simulink model "DOF4_model"  (R2022b)
settings: Solver=VariableStepAuto  StartTime=0.0  StopTime=10.0  RelTol=1e-3
values from neighbouring files (symbols this model uses):
  cdamper = 1500    [Quarter_car_model_parameters.m]
  F0 = 3924    [Quarter_car_model_parameters.m]
  g = 9.81    [Longitudinal_braking_parameters.m]    (also in Longitudinal_driving_parameters.m; Quarter_car_model_parameters.m)
  kspring = 35500    [Quarter_car_model_parameters.m]
  ktyre = 300000    [Quarter_car_model_parameters.m]
  ms = 400    [Quarter_car_model_parameters.m]
  mus = 30    [Quarter_car_model_parameters.m]
  z0tyre = (ms+mus) * g/ktyre    (= 0.014061)    [Quarter_car_model_parameters.m]
settings Model: Creator=webstert  LastModifiedBy=webstert

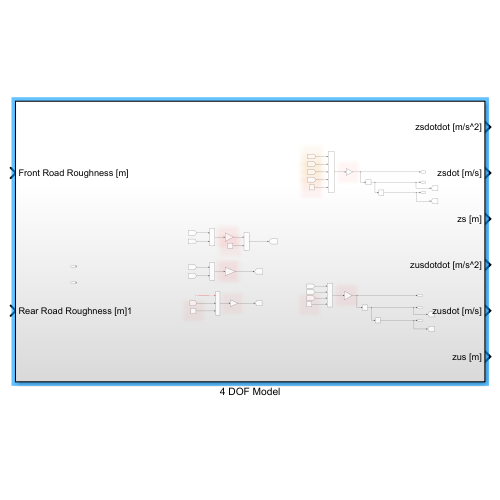
[thumbnail: Simulink's stored preview of the top-level diagram]
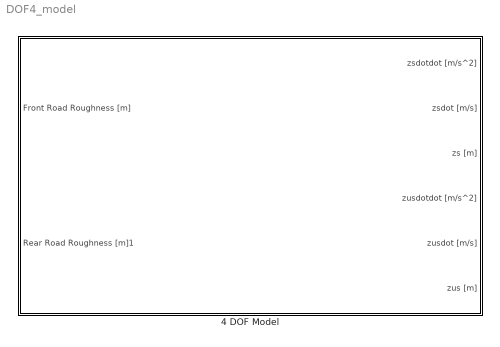
== system DOF4_model ==
  4 DOF Model : Subsystem

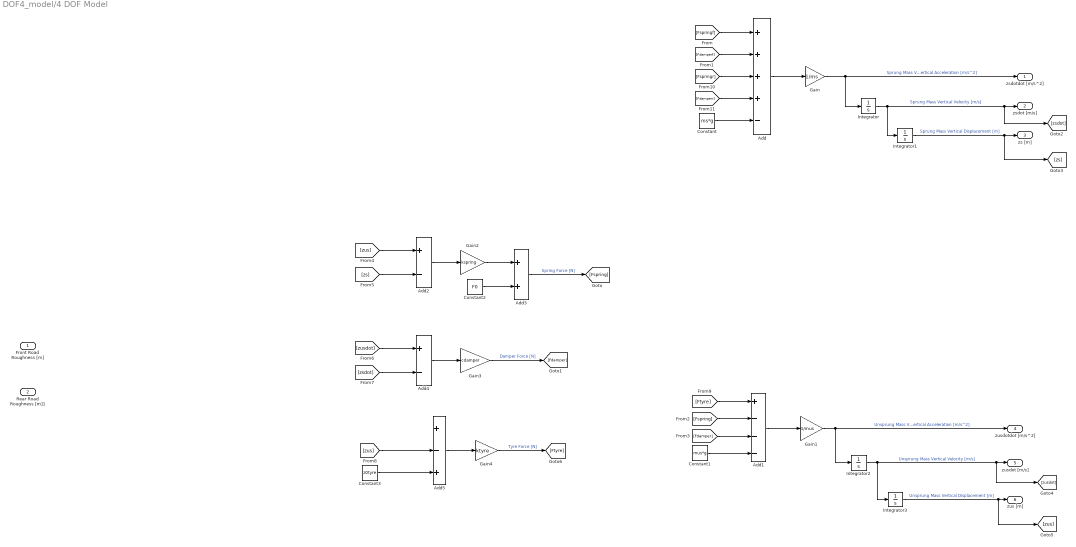
== system DOF4_model/4 DOF Model ==
  Front Road Roughness [m] : Inport
  Rear Road Roughness [m]1 : Inport  Port=2
  Add : Sum  Inputs=++++-
  Add1 : Sum  Inputs=+---
  Add2 : Sum  Inputs=+-
  Add3 : Sum
  Add4 : Sum  Inputs=+-
  Add5 : Sum  Inputs=+-+
  Constant : Constant  Value=ms*g
  Constant1 : Constant  Value=mus*g
  Constant2 : Constant  Value=F0
  Constant3 : Constant  Value=z0tyre
  Gain : Gain  Gain=1/ms
  Gain1 : Gain  Gain=1/mus
  Gain2 : Gain  Gain=kspring
  Gain3 : Gain  Gain=cdamper
  Gain4 : Gain  Gain=ktyre
  Integrator{,1..3} (4 alike) : Integrator
  zsdotdot [m/s^2] : Outport
  zsdot [m/s] : Outport  Port=2
  zs [m] : Outport  Port=3
  zusdotdot [m/s^2] : Outport  Port=4
  zusdot [m/s] : Outport  Port=5
  zus [m] : Outport  Port=6
  wires:
  [Fdamperf] -> Add/2
  [Fspringf] -> Add/1
  Gain4/1 -> [Ftyre]  "Tyre Force [N]"
  ? -> Add5/1
  [zusdot] -> Add4/1
  Constant3/1 -> Add5/3
  Add2/1 -> Gain2/1
  [zs] -> Add2/2
  Add5/1 -> Gain4/1
  Add1/1 -> Gain1/1
  Integrator3/1 -> [zus], zus [m]/1  "Unsprung Mass Vertical Displacement [m]"
  [Fdamper] -> Add1/3
  Gain1/1 -> zusdotdot [m/s^2]/1, Integrator2/1  "Unsprung Mass Vertical Acceleration [m/s^2]"
  Integrator1/1 -> [zs], zs [m]/1  "Sprung Mass Vertical Displacement [m]"
  Add4/1 -> Gain3/1
  Add3/1 -> [Fspring]  "Spring Force [N]"
  [Ftyre] -> Add1/1
  [Fspring] -> Add1/2
  Constant1/1 -> Add1/4
  [zsdot] -> Add4/2
  [zus] -> Add5/2
  Constant/1 -> Add/5
  Integrator/1 -> [zsdot], zsdot [m/s]/1, Integrator1/1  "Sprung Mass Vertical Velocity [m/s]"
  Gain2/1 -> Add3/1
  Constant2/1 -> Add3/2
  Add/1 -> Gain/1
  Gain/1 -> Integrator/1, zsdotdot [m/s^2]/1  "Sprung Mass Vertical Acceleration [m/s^2]"
  Integrator2/1 -> [zusdot], zusdot [m/s]/1, Integrator3/1  "Unsprung Mass Vertical Velocity [m/s]"
  Gain3/1 -> [Fdamper]  "Damper Force [N]"
  [zus] -> Add2/1
  [Fspringr] -> Add/3
  [Fdamperr] -> Add/4
